simulink library "simetranss"  (R2024b)
settings: Solver=VariableStepAuto  StartTime=0.0  StopTime=10.0  RelTol=1e-3
PostLoadFcn:
  | Ts=1e-6
InitFcn:
  | Ts=1e-6
undefined symbols (not defined in the file): C, C_601, C_603, C_606, CC, Csnu, Csnubber, DiscIntNeverNeededParam, DPL, DPL1ph, FluxTable, ft2km, gcbh, h, Half, Imap2, L, L_601, L_603, L_606, Lbase, LpejoSw, Newton, R_601, R_603, R_606, Raphson, ResistanceM, Roff, Ron, RotorAngles, Rsnu, Rsnubber, Rt4, SampleTime, simetran, sps, sps_rtmsupport, StatorCurrents, T_2wind_ratio, T_Lpu, T_Lpu_pri, T_Rpu, T_Rpu_pri, T_Vpri, T_Vpri_15comp, T_Vsec, Ti, Ts_Power, Z, Zbase, Zm
libraries: fl_lib x248, ee_lib x146, nesl_utility x122, $bdroot x29, simulink x15, eeGeneralControl x2, spsStairGeneratorLib x2, artemis x1
(part 9 of 12)

== system simetranss/Machines/MATE Induction Machine/Matrice ==
  we : Inport
  park : Inport  Port=2
  0 : Constant  Value=[0 0 0 0 0 0 0 0 0 0 0 ]
  1 : Constant  Value=[0 0]
  2 : Constant  Value=0
  3 : Constant  Value=[0 0 0 0 0 0 0 0 0 0 0 ]
  4 : Constant  Value=[0 0]
  5 : Constant  Value=0
  Divide4 : Product  Multiplication=Matrix(*)
  Gain1 : Gain  Gain=1/(Lr*Ls-Lm*Lm)
  Gain3 : Gain  Gain=-1
  Gain6 : Gain
  Gain7 : Gain
  Gain8 : Gain  Gain=-1
  L-1*discriminant : Constant  Value="[Lr 0 -Lm 0; 0 Lr 0 -Lm; -Lm 0  Ls  0;  0  -Lm  0  Ls]"
  Mux1 : Mux  Inputs=[11 1 2 1 1]
  Mux2 : Mux  Inputs=[1 1 2 1 11]
  R : Constant  Value="[-Rs 0 0 0; 0 -Rs 0 0; 0 0  -Rr  0;  0  0  0  -Rr]"
  Reshape2 : Reshape  OutputDimensionality=Customize  OutputDimensions=[4,4]
  Switch : Switch  Criteria=u2 > Threshold  Threshold=0.5  SaturateOnIntegerOverflow=off  InputSameDT=off
  Adq : Outport  VectorParamsAs1DForOutWhenUnconnected=off
  invLdq : Outport  Port=2  VectorParamsAs1DForOutWhenUnconnected=off
  speed term : Outport  Port=3  VectorParamsAs1DForOutWhenUnconnected=off
  wires:
  L-1*discriminant/1 -> Gain1/1
  Reshape2/1 -> speed term/1  "OMEGA"
  R/1 -> Divide4/1
  Gain7/1 -> Mux1/2
  2/1 -> Mux1/5
  1/1 -> Mux1/3
  Divide4/1 -> Adq/1
  Gain3/1 -> Mux1/4
  0/1 -> Mux1/1
  Gain1/1 -> Divide4/2, invLdq/1  "inv(L)"
  Gain8/1 -> Mux2/2
  4/1 -> Mux2/3
  Gain6/1 -> Mux2/4
  we/1 -> Gain6/1, Gain8/1, Gain7/1, Gain3/1
  park/1 -> Switch/2
  Switch/1 -> Reshape2/1
  Mux1/1 -> Switch/1
  Mux2/1 -> Switch/3
  5/1 -> Mux2/1
  3/1 -> Mux2/5

== system simetranss/Machines/MATE Induction Machine/choose ==
  In1 : Inport
  In2 : Inport  Port=2
  In3 : Inport  Port=3
  In4 : Inport  Port=4
  In5 : Inport  Port=5
  In6 : Inport  Port=6
  In7 : Inport  Port=7
  In8 : Inport  Port=8
  In9 : Inport  Port=9
  In10 : Inport  Port=10
  Constant6 : Constant  Value=park_num
  Switch{1..5} (5 alike) : Switch  Criteria=u2 > Threshold  Threshold=0.5  SaturateOnIntegerOverflow=off  InputSameDT=off
  Out1 : Outport
  Out2 : Outport  Port=2
  Out3 : Outport  Port=3
  Out4 : Outport  Port=4
  Out5 : Outport  Port=5
  wires:
  Switch5/1 -> Out5/1
  In7/1 -> Switch2/3
  Switch4/1 -> Out4/1
  In10/1 -> Switch5/3
  In3/1 -> Switch3/1
  In5/1 -> Switch5/1
  In8/1 -> Switch3/3
  In2/1 -> Switch2/1
  In1/1 -> Switch1/1
  In6/1 -> Switch1/3
  In4/1 -> Switch4/1
  Switch2/1 -> Out2/1
  In9/1 -> Switch4/3
  Constant6/1 -> Switch1/2, Switch2/2, Switch3/2, Switch4/2, Switch5/2
  Switch1/1 -> Out1/1
  Switch3/1 -> Out3/1

== system simetranss/Machines/MATE Induction Machine/dq_fixedTransform ==
  note: Fixed reference frame
      | like rotor reference but with constant angle input=0
  Constant1 : Constant  Value=[1 -0.5 -0.5;0 sqrt(3)/2 -sqrt(3)/2]
  Gain1 : Gain  Gain=sqrt(2/3)
  Tstator : Outport  VectorParamsAs1DForOutWhenUnconnected=off
  wires:
  Constant1/1 -> Gain1/1
  Gain1/1 -> Tstator/1

== system simetranss/Machines/MATE Induction Machine/dq_rotortransform ==
  note: (rotor dq transformation reference frame)
  angle : Inport
  Enable : EnablePort
  Constant2 : Constant  Value=[1 -0.5 -0.5;0 sqrt(3)/2 -sqrt(3)/2]
  Divide : Product  Multiplication=Matrix(*)
  Gain2 : Gain  Gain=-1
  Gain4 : Gain  Gain=sqrt(2/3)
  Mux6 : Mux
  Reshape4 : Reshape  OutputDimensionality=Customize  OutputDimensions=[2,2]
  Trigonometric Function1 : Trigonometry  Operator=cos
  Trigonometric Function2 : Trigonometry
  Trotor : Outport  VectorParamsAs1DForOutWhenUnconnected=off
  wires:
  Gain4/1 -> Trotor/1  "T"
  angle/1 -> Trigonometric Function1/1, Trigonometric Function2/1
  Trigonometric Function1/1 -> Mux6/1, Mux6/4
  Trigonometric Function2/1 -> Gain2/1, Mux6/3
  Mux6/1 -> Reshape4/1
  Reshape4/1 -> Divide/1
  Constant2/1 -> Divide/2
  Divide/1 -> Gain4/1
  Gain2/1 -> Mux6/2

== system simetranss/Machines/MATE Permanent Magnet Machine (ALT1)/1 step prediction5 ==
  In1 : Inport
  Gain2 : Gain  Gain=2
  Gain3 : Gain  Gain=-1
  Sum5 : Sum  SaturateOnIntegerOverflow=on
  Unit Delay1 : UnitDelay  SampleTime=Ts  HasFrameUpgradeWarning=on
  Out1 : Outport  VectorParamsAs1DForOutWhenUnconnected=off
  wires:
  Unit Delay1/1 -> Gain3/1
  Gain2/1 -> Sum5/1
  Gain3/1 -> Sum5/2
  In1/1 -> Gain2/1, Unit Delay1/1
  Sum5/1 -> Out1/1

== system simetranss/Machines/MATE Permanent Magnet Machine (ALT1)/ABC<->dq ==
  note: (rotor dq transformation reference frame)
  angle : Inport
  Constant2 : Constant  Value=[1 -0.5 -0.5;0 sqrt(3)/2 -sqrt(3)/2]
  Divide : Product  Multiplication=Matrix(*)
  Gain2 : Gain  Gain=-1
  Gain4 : Gain  Gain=sqrt(2/3)
  Mux6 : Mux
  Reshape4 : Reshape  OutputDimensionality=Customize  OutputDimensions=[2,2]
  Trigonometric Function1 : Trigonometry  Operator=cos
  Trigonometric Function2 : Trigonometry
  T : Outport  VectorParamsAs1DForOutWhenUnconnected=off
  wires:
  Gain2/1 -> Mux6/2
  Divide/1 -> Gain4/1
  Constant2/1 -> Divide/2
  Reshape4/1 -> Divide/1
  Mux6/1 -> Reshape4/1
  Trigonometric Function2/1 -> Mux6/3, Gain2/1
  Trigonometric Function1/1 -> Mux6/4, Mux6/1
  angle/1 -> Trigonometric Function2/1, Trigonometric Function1/1
  Gain4/1 -> T/1  "T"

== system simetranss/Machines/MATE Permanent Magnet Machine (ALT1)/Bd ==
  Bc : Inport
  Product1 : Product  Multiplication=Matrix(*)  SaturateOnIntegerOverflow=on  OutDataTypeStr=Inherit: Same as first input
  trapeze has Ts/2 factor on B : Gain  Gain=Ts/2  SaturateOnIntegerOverflow=on  OutDataTypeStr=Inherit: Same as input  ParamDataTypeStr=Inherit: Same as input
  u1 : Constant  Value=Aden
  Bd : Outport  VectorParamsAs1DForOutWhenUnconnected=off
  wires:
  u1/1 -> Product1/1
  Bc/1 -> trapeze has Ts/2 factor on B/1
  trapeze has Ts/2 factor on B/1 -> Product1/2
  Product1/1 -> Bd/1

== system simetranss/Machines/MATE Permanent Magnet Machine (ALT1)/PMSM equations ==
  note: phiTot contains magnet flux
  Ad : Inport
  Bd : Inport  Port=2
  C : Inport  Port=3
  Bd_sp_term : Inport  Port=4
  C1 : Inport  Port=5
  u[n+1] : Inport  Port=6
  u_speedterm : Inport  Port=7
  fluxmagnet : Inport  Port=8
  flux_del : Inport  Port=9
  Product{1,3,5..6,8} (5 alike) : Product  Multiplication=Matrix(*)  SaturateOnIntegerOverflow=on  OutDataTypeStr=Inherit: Same as first input
  Sum1 : Sum  SaturateOnIntegerOverflow=on
  Sum2 : Sum  Inputs=+++  SaturateOnIntegerOverflow=on
  Sum3 : Sum  SaturateOnIntegerOverflow=on
  Sum5 : Sum  SaturateOnIntegerOverflow=on
  z-1 : UnitDelay  SampleTime=Ts  HasFrameUpgradeWarning=on
  z-2 : UnitDelay  SampleTime=Ts  HasFrameUpgradeWarning=on
  Ihist : Outport  VectorParamsAs1DForOutWhenUnconnected=off
  phi[n+1] : Outport  Port=2  VectorParamsAs1DForOutWhenUnconnected=off
  phiTot : Outport  Port=3  VectorParamsAs1DForOutWhenUnconnected=off
  wires:
  Bd/1 -> z-2/1
  C/1 -> Product6/1
  Product5/1 -> Sum3/1, Sum2/1
  Sum2/1 -> Product6/2, z-1/1  "Ad*phi[n]+Bd*u[n]"
  Ad/1 -> Product3/1
  u[n+1]/1 -> Product5/2
  Product3/1 -> Sum2/2
  z-1/1 -> Sum3/2
  z-2/1 -> Product5/1
  u_speedterm/1 -> Product8/2
  Bd_sp_term/1 -> Product8/1
  Product8/1 -> Sum2/3
  fluxmagnet/1 -> Sum5/2
  Sum5/1 -> phiTot/1
  Sum3/1 -> Sum5/1, phi[n+1]/1, Product3/2  "new_x"
  Product6/1 -> Sum1/1
  Sum1/1 -> Ihist/1
  Product1/1 -> Sum1/2
  C1/1 -> Product1/1
  flux_del/1 -> Product1/2

== system simetranss/Machines/MATE Permanent Magnet Machine (ALT1)/omega ==
  note: Produces: OMEGA=
      | [ 0  w ;
      | -w  0]
  In1 : Inport
  1 : Constant  Value=0
  Gain1 : Gain  Gain=-1
  Mux1 : Mux
  Reshape2 : Reshape  OutputDimensionality=Customize  OutputDimensions=[2,2]
  OMEGA : Outport
  wires:
  Reshape2/1 -> OMEGA/1  "OMEGA"
  Gain1/1 -> Mux1/2
  1/1 -> Mux1/1, Mux1/4
  Mux1/1 -> Reshape2/1
  In1/1 -> Mux1/3, Gain1/1

== system simetranss/Machines/MATE Permanent Magnet Synchronous Machine/ABC<->dq ==
  note: test for reorder block
  note: (rotor dq transformation reference frame)
  note: Derivative
  angle : Inport
  we : Inport  Port=2
  Constant : Constant  Commented=on
  Constant1 : Constant  Commented=on  Value=2
  Constant2 : Constant  Value=[1 -0.5 -0.5;0 sqrt(3)/2 -sqrt(3)/2]
  Constant3 : Constant  Commented=on  Value=3
  Constant4 : Constant  Commented=on  Value=4
  Display : Display  Commented=on
  Divide : Product  Multiplication=Matrix(*)
  Divide1 : Product  Multiplication=Matrix(*)
  Divide2 : Product
  Gain1 : Gain  Gain=sqrt(2/3)
  Gain2 : Gain  Gain=-1
  Gain3 : Gain  Gain=-1
  Gain4 : Gain  Gain=sqrt(2/3)
  Math Function3 : Math  Operator=transpose  SignedPower=on
  Mux1 : Mux
  Mux2 : Mux  Commented=on
  Mux6 : Mux
  Reshape1 : Reshape  OutputDimensionality=Customize  OutputDimensions=[2,2]
  Reshape2 : Reshape  Commented=on  OutputDimensionality=Customize  OutputDimensions=[2,2]
  Reshape4 : Reshape  OutputDimensionality=Customize  OutputDimensions=[2,2]
  Trigonometric Function1 : Trigonometry  Operator=cos
  Trigonometric Function2 : Trigonometry
  T : Outport  VectorParamsAs1DForOutWhenUnconnected=off
  dT-1/dt : Outport  Port=2  VectorParamsAs1DForOutWhenUnconnected=off
  wires:
  Reshape2/1 -> Display/1
  Mux2/1 -> Reshape2/1
  Constant4/1 -> Mux2/4
  Constant3/1 -> Mux2/3
  Constant1/1 -> Mux2/2
  Constant/1 -> Mux2/1
  we/1 -> Divide2/2
  Divide2/1 -> Gain1/1
  Divide1/1 -> Divide2/1
  Gain1/1 -> dT-1/dt/1  "T"
  Reshape1/1 -> Divide1/2
  Math Function3/1 -> Divide1/1
  Mux1/1 -> Reshape1/1
  Gain3/1 -> Mux1/3
  Gain2/1 -> Mux6/2, Mux1/4, Mux1/1  "-sin"
  Divide/1 -> Gain4/1
  Constant2/1 -> Divide/2, Math Function3/1
  Reshape4/1 -> Divide/1
  Mux6/1 -> Reshape4/1
  Trigonometric Function2/1 -> Mux6/3, Gain2/1
  Trigonometric Function1/1 -> Mux6/4, Mux6/1, Mux1/2, Gain3/1  "cos"
  angle/1 -> Trigonometric Function2/1, Trigonometric Function1/1
  Gain4/1 -> T/1  "T"

== system simetranss/Machines/MATE Synchronous Machine/1 step prediction1 ==
  In1 : Inport
  Gain2 : Gain  Gain=2
  Gain3 : Gain  Gain=-1
  Sum5 : Sum  SaturateOnIntegerOverflow=on
  Unit Delay1 : UnitDelay  SampleTime=Ts  HasFrameUpgradeWarning=on
  Out1 : Outport
  wires:
  Unit Delay1/1 -> Gain3/1
  Gain2/1 -> Sum5/1
  Gain3/1 -> Sum5/2
  In1/1 -> Gain2/1, Unit Delay1/1
  Sum5/1 -> Out1/1

== system simetranss/Machines/MATE Synchronous Machine/1 step prediction2 ==
  In1 : Inport
  Gain2 : Gain  Gain=2
  Gain3 : Gain  Gain=-1
  Sum5 : Sum  SaturateOnIntegerOverflow=on
  Unit Delay1 : UnitDelay  SampleTime=Ts  HasFrameUpgradeWarning=on
  Out1 : Outport
  wires:
  Sum5/1 -> Out1/1
  In1/1 -> Unit Delay1/1, Gain2/1
  Gain3/1 -> Sum5/2
  Gain2/1 -> Sum5/1
  Unit Delay1/1 -> Gain3/1

== system simetranss/Machines/MATE Synchronous Machine/ABC<->0 ==
  note: (homopolar transform)
  Constant2 : Constant  Value=[1 1 1]  VectorParams1D=off
  Gain4 : Gain  Gain=sqrt(1/3)
  T0 : Outport
  wires:
  Constant2/1 -> Gain4/1
  Gain4/1 -> T0/1  "T"

== system simetranss/Machines/MATE Synchronous Machine/ABC<->dq ==
  note: The Feild turn ratio gain has been moved directly in the Vfeild et IFeild signals
  note: (rotor dq transformation reference frame)
  angle : Inport
  Constant1 : Constant  Value="[0  ;0 ]"  VectorParams1D=off
  Constant2 : Constant  Value=[1 -0.5 -0.5;0 sqrt(3)/2 -sqrt(3)/2]
  Constant3 : Constant  Value=[0 0 0 Ns_on_Nf*0+1; 0 0 0 0 ; 0 0 0 0; 0 0 0 0]  VectorParams1D=off
  Divide : Product  Multiplication=Matrix(*)
  Gain2 : Gain  Gain=-1
  Gain4 : Gain  Gain=sqrt(2/3)
  Matrix Concatenate : Concatenate  Mode=Multidimensional array  ConcatenateDimension=2
  Matrix Concatenate1 : Concatenate  Mode=Multidimensional array
  Mux6 : Mux
  Reshape4 : Reshape  OutputDimensionality=Customize  OutputDimensions=[2,2]
  Selector : Selector  NumberOfDimensions=2  InputPortWidth=3  IndexOptions=Index vector (dialog),Index vector (dialog)  Indices=[1:nb_row-2],[1:4]  OutputSizes=1,1
  Trigonometric Function1 : Trigonometry  Operator=cos
  Trigonometric Function2 : Trigonometry
  T : Outport
  Tv : Outport  Port=2
  wires:
  Selector/1 -> Matrix Concatenate1/2
  angle/1 -> Trigonometric Function2/1, Trigonometric Function1/1
  Matrix Concatenate1/1 -> T/1
  Constant3/1 -> Selector/1
  Matrix Concatenate/1 -> Matrix Concatenate1/1
  Constant1/1 -> Matrix Concatenate/2
  Gain2/1 -> Mux6/2
  Divide/1 -> Gain4/1
  Constant2/1 -> Divide/2
  Reshape4/1 -> Divide/1
  Mux6/1 -> Reshape4/1
  Trigonometric Function2/1 -> Mux6/3, Gain2/1
  Trigonometric Function1/1 -> Mux6/4, Mux6/1
  Gain4/1 -> Matrix Concatenate/1, Tv/1  "T"

== system simetranss/Machines/MATE Synchronous Machine/Delta angle ==
  Vd : Inport  PortDimensions=1
  Vq : Inport  Port=2  PortDimensions=1
  Cartesian to Polar : Subsystem  mask(Cart2Polar){}
      mask help:
      | Transformation from cartesian to polar coordinates.
      | [x, y] -> [r, theta]
      |
      | r = sqrt(x^2 + y^2);
      | theta = atan(y/x);
      mask Help: Unmask this block for more help.
      mask Display: plot(0,0,100,100,[24,20,15,20,20],[85,95,85,95,20],[80,20,95,85,95,85],[70,20,20,15,20,24],[56,56,55,52,50,46],[20,26,31,35,38,42])
  Radians to Degrees : Subsystem  mask(RadiansToDegrees){}
      mask help:
      | Conversion from Radians to Degrees.
      |
      | D=180/pi*R
      mask Help: This block converts from Radians to Degrees.
      mask Display: disp('R2D')
  Terminator2 : Terminator
  delta : Outport
  wires:
  Cartesian to Polar/2(theta) -> Radians to Degrees/1(Radians in)
  Cartesian to Polar/1(r) -> Terminator2/1
  Vq/1 -> Cartesian to Polar/1(x)
  Radians to Degrees/1(Degrees out) -> delta/1  "delta"
  Vd/1 -> Cartesian to Polar/2(y)

== system simetranss/Machines/MATE Synchronous Machine/Electromagnetic Torque ==
  note: Te=phids*Iqs - phiqs*Ids
  note: Te computed from stator fluxes and currents
  phid_phiq : Inport
  id_iq : Inport  Port=2
  1-2 : Gain  Gain=[1 -1]
  Dot Product : DotProduct  OutDataTypeStr=Inherit: Inherit via internal rule
  Selector2 : Selector  InputPortWidth=2  IndexOptions=Index vector (dialog)  Indices="[2  1]"  OutputSizes=1
  Te : Outport
  wires:
  1-2/1 -> Dot Product/1
  Dot Product/1 -> Te/1
  phid_phiq/1 -> 1-2/1  "phids phiqs"
  Selector2/1 -> Dot Product/2  "iqs ids"
  id_iq/1 -> Selector2/1

== system simetranss/Machines/MATE Synchronous Machine/Phimqd ==
  note: Lad
  note: Laq
  note: phimq=  phiqs*(Laq/Ll)   +phikq1*(Laq/Llkq1)  +phikq2*(Laq/Llkq2)
      | phimd=  phids*(Lad/Ll)   +phifd*(Lad/Llfd)  + phikd*(Lad/Llkd)
  phi : Inport
  Laq : Inport  Port=2
  Lad : Inport  Port=3
  sat : Inport  Port=4
  1/Ll_d : Gain  Gain="[1/Lls   1/Llf 1/Llkd ]"  SaturateOnIntegerOverflow=on  OutDataTypeStr=Inherit: Same as input  ParamDataTypeStr=Inherit: Same as input
  1/Ll_q : Gain  Gain=[1/Lls 1/Llkq 1/Llkq2]  SaturateOnIntegerOverflow=on  OutDataTypeStr=Inherit: Same as input  ParamDataTypeStr=Inherit: Same as input
  Constant2 : Constant  Value=Lad
  Constant4 : Constant  Value=Laq
  Mux1 : Mux  Inputs=2
  Product1 : Product  RndMeth=Zero
  Product3 : Product  RndMeth=Zero
  Switch : Switch  Threshold=0.5  SaturateOnIntegerOverflow=off  InputSameDT=off
  Switch1 : Switch  Threshold=0.5  SaturateOnIntegerOverflow=off  InputSameDT=off
  "phid phifd phikd " : Selector  InputPortWidth=7  IndexOptions=Index vector (dialog)  Indices=[1 3 4]  OutputSizes=1
  phiq phikq1 (phikq2) : Selector  InputPortWidth=7  IndexOptions=Index vector (dialog)  Indices=[2 5 6]  OutputSizes=1
  sum : Sum  Inputs=+  InputSameDT=on  SaturateOnIntegerOverflow=on  OutDataTypeStr=Inherit: Same as first input
  sum1 : Sum  Inputs=+  InputSameDT=on  SaturateOnIntegerOverflow=on  OutDataTypeStr=Inherit: Same as first input
  phim_dq : Outport
  wires:
  Product1/1 -> Mux1/2  "phim_q"
  Product3/1 -> Mux1/1  "phim_d"
  "phid phifd phikd "/1 -> 1/Ll_d/1
  1/Ll_q/1 -> sum/1
  phiq phikq1 (phikq2)/1 -> 1/Ll_q/1
  phi/1 -> phiq phikq1 (phikq2)/1, "phid phifd phikd "/1
  1/Ll_d/1 -> sum1/1
  Mux1/1 -> phim_dq/1
  sum/1 -> Product1/2  "phimq"
  sum1/1 -> Product3/1  "phimd"
  Switch/1 -> Product1/1
  sat/1 -> Switch1/2, Switch/2
  Constant4/1 -> Switch/3
  Laq/1 -> Switch/1
  Constant2/1 -> Switch1/3
  Lad/1 -> Switch1/1
  Switch1/1 -> Product3/2

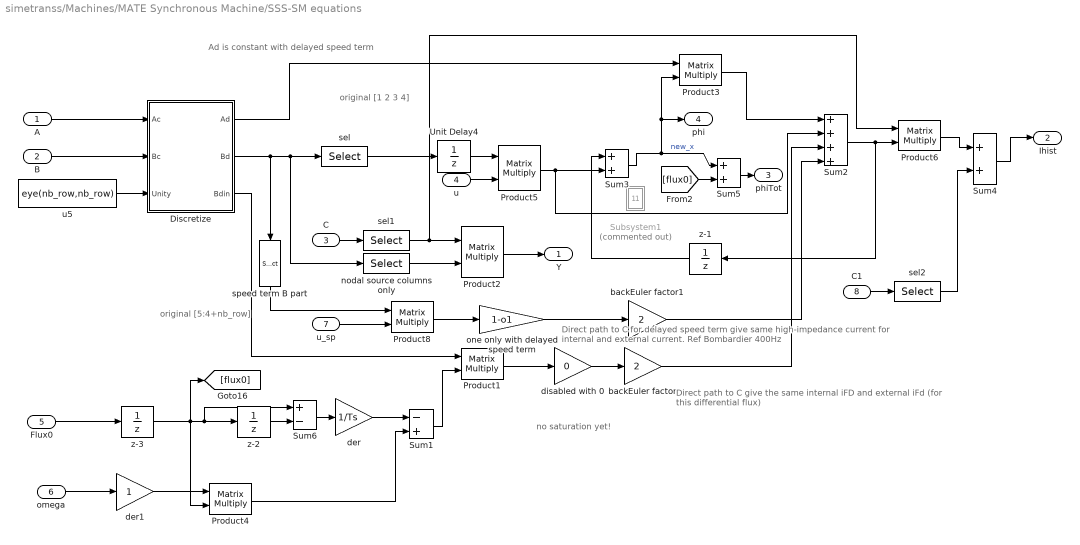
== system simetranss/Machines/MATE Synchronous Machine/SSS-SM equations ==
  note: no saturation yet!
  note: original
      | [1 2 3  4]
  note: original
      | [5:4+nb_row]
  note: Ad is constant with delayed speed term
  note: Direct path to C for delayed speed term give same high-impedance current
      | for internal and external current. Ref Bombardier 400Hz
  note: Direct path to C give the same internal iFD and external iFd
      | (for this differential flux)
  A : Inport
  B : Inport  Port=2
  C : Inport  Port=3
  u : Inport  Port=4
  Flux0 : Inport  Port=5
  omega : Inport  Port=6
  u_sp : Inport  Port=7
  C1 : Inport  Port=8
  Discretize : Subsystem
  Product{1..6,8} (7 alike) : Product  Multiplication=Matrix(*)  SaturateOnIntegerOverflow=on  OutDataTypeStr=Inherit: Same as first input
  Subsystem1 : Subsystem  Commented=on
  Sum1 : Sum  Inputs=-+  SaturateOnIntegerOverflow=on
  Sum2 : Sum  Inputs=++++  SaturateOnIntegerOverflow=on
  Sum3 : Sum  SaturateOnIntegerOverflow=on
  Sum4 : Sum  Inputs=2  SaturateOnIntegerOverflow=on
  Sum5 : Sum  SaturateOnIntegerOverflow=on
  Sum6 : Sum  Inputs=+-  SaturateOnIntegerOverflow=on
  Unit Delay4 : UnitDelay  SampleTime=Ts  HasFrameUpgradeWarning=on
  backEuler factor : Gain  Gain=2  SaturateOnIntegerOverflow=on  OutDataTypeStr=Inherit: Same as input  ParamDataTypeStr=Inherit: Same as input
  backEuler factor1 : Gain  Gain=2  SaturateOnIntegerOverflow=on  OutDataTypeStr=Inherit: Same as input  ParamDataTypeStr=Inherit: Same as input
  der : Gain  Gain=1/Ts  SaturateOnIntegerOverflow=on  OutDataTypeStr=Inherit: Same as input  ParamDataTypeStr=Inherit: Same as input
  der1 : Gain  SaturateOnIntegerOverflow=on  OutDataTypeStr=Inherit: Same as input  ParamDataTypeStr=Inherit: Same as input
  disabled with 0 : Gain  Gain=0  SaturateOnIntegerOverflow=on  OutDataTypeStr=Inherit: Same as input  ParamDataTypeStr=Inherit: Same as input
  nodal source columns only : Selector  NumberOfDimensions=2  InputPortWidth=3  IndexOptions=Index vector (dialog),Index vector (dialog)  Indices=[1:nb_row],[1 2 3]  OutputSizes=1,1
  one only with delayed speed term : Gain  Gain=1-o1
  sel : Selector  NumberOfDimensions=2  InputPortWidth=3  IndexOptions=Index vector (dialog),Index vector (dialog)  Indices="[1:nb_row],[1 2 3  ]"  OutputSizes=1,1
  sel1 : Selector  NumberOfDimensions=2  InputPortWidth=3  IndexOptions=Index vector (dialog),Index vector (dialog)  Indices=[1 2 3 ],[1:nb_row]  OutputSizes=1,1
  sel2 : Selector  InputPortWidth=4  IndexOptions=Index vector (dialog)  Indices=[1 2 3 ]  OutputSizes=1
  speed term B part : Selector  NumberOfDimensions=2  InputPortWidth=3  IndexOptions=Index vector (dialog),Index vector (dialog)  Indices=[1:nb_row],[4:3+nb_row+1]  OutputSizes=1,1
  u5 : Constant  Value=eye(nb_row,nb_row)
  z-1 : UnitDelay  InitialCondition=flux_0  SampleTime=Ts  HasFrameUpgradeWarning=on
  z-2 : UnitDelay  SampleTime=Ts  HasFrameUpgradeWarning=on
  z-3 : UnitDelay  SampleTime=Ts  HasFrameUpgradeWarning=on
  Y : Outport
  Ihist : Outport  Port=2
  phiTot : Outport  Port=3
  phi : Outport  Port=4
  wires:
  backEuler factor1/1 -> Sum2/4
  one only with delayed speed term/1 -> backEuler factor1/1
  Product8/1 -> one only with delayed speed term/1
  speed term B part/1 -> Product8/1
  u_sp/1 -> Product8/2
  sel/1 -> Unit Delay4/1
  Unit Delay4/1 -> Product5/1
  backEuler factor/1 -> Sum2/3
  Sum1/1 -> Product1/2
  der1/1 -> Product4/1
  [flux0] -> Sum5/2
  der/1 -> Sum1/1
  Product4/1 -> Sum1/2
  omega/1 -> der1/1
  Discretize/3(Bdin) -> Product1/1
  z-3/1 -> Product4/2, [flux0], Sum6/1, z-2/1
  Sum6/1 -> der/1
  z-2/1 -> Sum6/2
  Sum5/1 -> phiTot/1
  Flux0/1 -> z-3/1
  Discretize/2(Bd) -> speed term B part/1, sel/1, nodal source columns only/1
  u/1 -> Product5/2
  Discretize/1(Ad) -> Product3/1
  Sum2/1 -> Product6/2, z-1/1
  Sum3/1 -> Product3/2, phi/1, Sum5/1  "new_x"
  Product3/1 -> Sum2/1
  Product5/1 -> Sum3/2, Sum2/2
  C/1 -> sel1/1
  B/1 -> Discretize/2(Bc)
  A/1 -> Discretize/1(Ac)
  Product2/1 -> Y/1
  u5/1 -> Discretize/3(Unity)
  nodal source columns only/1 -> Product2/2
  sel1/1 -> Product6/1, Product2/1
  C1/1 -> sel2/1
  Product6/1 -> Sum4/1
  Sum4/1 -> Ihist/1
  sel2/1 -> Sum4/2
  z-1/1 -> Sum3/1
  Product1/1 -> disabled with 0/1
  disabled with 0/1 -> backEuler factor/1

== system simetranss/Machines/MATE Synchronous Machine/SSS-SM equations zero sequence only ==
  A : Inport
  B : Inport  Port=2
  C : Inport  Port=3
  u : Inport  Port=4
  Discretize : Subsystem
  Product{2..3,5..6} (4 alike) : Product  Multiplication=Matrix(*)  SaturateOnIntegerOverflow=on  OutDataTypeStr=Inherit: Same as first input
  Sum2 : Sum  SaturateOnIntegerOverflow=on
  Sum3 : Sum  SaturateOnIntegerOverflow=on
  u5 : Constant
  z-1 : UnitDelay  SampleTime=Ts  HasFrameUpgradeWarning=on
  Y0 : Outport
  Ihist0 : Outport  Port=2
  phi0 : Outport  Port=3
  wires:
  Discretize/2(Bd) -> Product2/2, Product5/1
  z-1/1 -> Sum3/1
  u/1 -> Product5/2
  Discretize/1(Ad) -> Product3/1
  Sum2/1 -> Product6/2, z-1/1
  Sum3/1 -> phi0/1, Product3/2  "new_x"
  Product3/1 -> Sum2/1
  Product5/1 -> Sum3/2, Sum2/2
  Product6/1 -> Ihist0/1
  C/1 -> Product2/1, Product6/1
  B/1 -> Discretize/2(Bc)
  A/1 -> Discretize/1(Ac)
  Product2/1 -> Y0/1
  u5/1 -> Discretize/3(Unity)

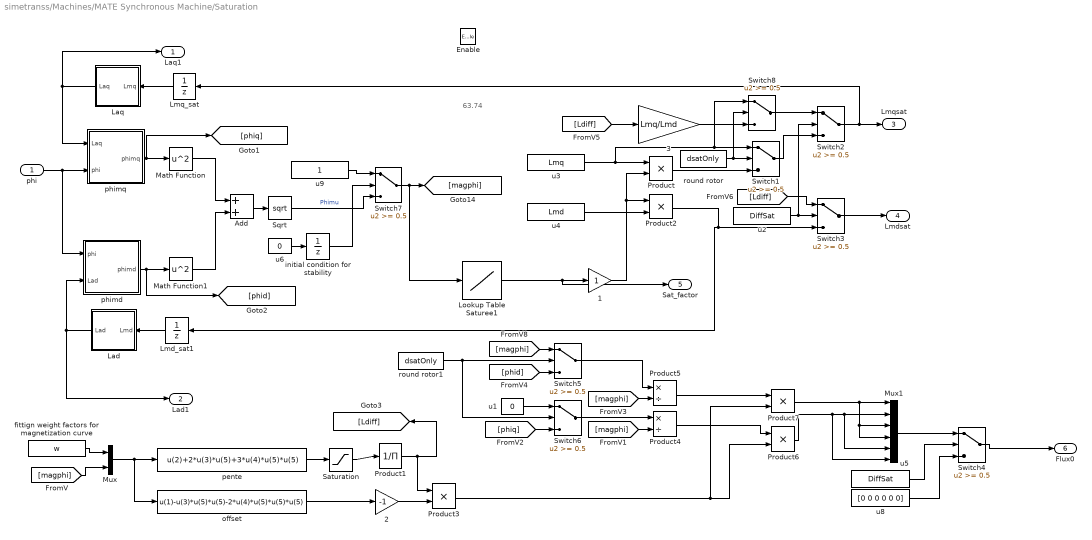
== system simetranss/Machines/MATE Synchronous Machine/Saturation ==
  note: 63.74
  phi : Inport
  Enable : EnablePort
  1 : Gain  SaturateOnIntegerOverflow=on  OutDataTypeStr=Inherit: Same as input  ParamDataTypeStr=Inherit: Same as input
  2 : Gain  Gain=-1  SaturateOnIntegerOverflow=on  OutDataTypeStr=Inherit: Same as input  ParamDataTypeStr=Inherit: Same as input
  3 : Gain  Gain=Lmq/Lmd  SaturateOnIntegerOverflow=on  OutDataTypeStr=Inherit: Same as input  ParamDataTypeStr=Inherit: Same as input
  Add : Sum
  Lad : Subsystem
  Laq : Subsystem
  Lmd_sat1 : UnitDelay  InitialCondition=Lmd  SampleTime=Ts  HasFrameUpgradeWarning=on
  Lmq_sat : UnitDelay  InitialCondition=Lmq  SampleTime=Ts  HasFrameUpgradeWarning=on
  Lookup Table Saturee1 : Lookup  InputValues=table_flux_input  Table=table_saturation_factor  SaturateOnIntegerOverflow=off
  Math Function : Math  Operator=square  SignedPower=on
  Math Function1 : Math  Operator=square  SignedPower=on
  Mux : Mux  Inputs=2
  Mux1 : Mux  Inputs=6
  Product{,2..3,6..7} (5 alike) : Product  RndMeth=Zero
  Product1 : Product  Inputs=/  RndMeth=Zero
  Product4 : Product  Inputs=*/  RndMeth=Zero
  Product5 : Product  Inputs=*/  RndMeth=Zero
  Saturation : Saturate  UpperLimit=inf  LowerLimit=1e-7
  Sqrt : Sqrt  OutputSignalType=real
  Switch{1..8} (8 alike) : Switch  Threshold=0.5  SaturateOnIntegerOverflow=off  InputSameDT=off
  fittign weight factors for magnetization curve : Constant  Value=w
  initial condition for stability : UnitDelay  InitialCondition=1  SampleTime=Ts  HasFrameUpgradeWarning=on
  offset : Fcn  Expr=u(1)-u(3)*u(5)*u(5)-2*u(4)*u(5)*u(5)*u(5)
  pente : Fcn  Expr=u(2)+2*u(3)*u(5)+3*u(4)*u(5)*u(5)
  phimd : Subsystem
  phimq : Subsystem
  round rotor : Constant  Value=dsatOnly
  round rotor1 : Constant  Value=dsatOnly
  u1 : Constant  Value=0
  u2 : Constant  Value=DiffSat
  u3 : Constant  Value=Lmq
  u4 : Constant  Value=Lmd
  u5 : Constant  Value=DiffSat
  u6 : Constant  Value=0
  u8 : Constant  Value=[0 0 0 0 0 0]
  u9 : Constant
  Laq1 : Outport
  Lad1 : Outport  Port=2
  Lmqsat : Outport  Port=3
  Lmdsat : Outport  Port=4
  Sat_factor : Outport  Port=5
  Flux0 : Outport  Port=6
  wires:
  3/1 -> Switch8/3
  Switch8/1 -> Switch2/1
  round rotor1/1 -> Switch5/2, Switch6/2
  u1/1 -> Switch6/1
  [magphi] -> Switch5/1
  Switch6/1 -> Product4/1
  Switch5/1 -> Product5/1
  [phiq] -> Switch6/3
  [phid] -> Switch5/3
  initial condition for stability/1 -> Switch7/2
  Switch7/1 -> Lookup Table Saturee1/1, [magphi]
  u9/1 -> Switch7/1
  Saturation/1 -> Product1/1
  pente/1 -> Saturation/1
  u8/1 -> Switch4/3
  u5/1 -> Switch4/2
  Switch4/1 -> Flux0/1
  Mux1/1 -> Switch4/1
  [Ldiff] -> Switch3/1
  [Ldiff] -> 3/1
  u2/1 -> Switch2/2, Switch3/2
  Switch2/1 -> Lmqsat/1, Lmq_sat/1
  Switch3/1 -> Lmdsat/1
  Product4/1 -> Product6/1
  Product5/1 -> Product7/1
  Product7/1 -> Mux1/4, Mux1/3, Mux1/1
  Product6/1 -> Mux1/6, Mux1/5, Mux1/2
  [magphi] -> Product5/2
  [magphi] -> Product4/2
  Product3/1 -> Product6/2, Product7/2
  2/1 -> Product3/2
  offset/1 -> 2/1
  Product1/1 -> Product3/1, [Ldiff]
  Mux/1 -> offset/1, pente/1
  [magphi] -> Mux/2
  fittign weight factors for magnetization curve/1 -> Mux/1
  Lookup Table Saturee1/1 -> Sat_factor/1, 1/1
  1/1 -> Product2/1, Product/2
  Switch1/1 -> Switch2/3
  Product/1 -> Switch1/3
  round rotor/1 -> Switch8/2, Switch1/2
  Lmq_sat/1 -> Laq/1(Lmq)
  phimq/1(phimq) -> Math Function/1, [phiq]
  Laq/1(Laq) -> Laq1/1, phimq/1(Laq)
  Lmd_sat1/1 -> Lad/1(Lmd)
  phimd/1(phimd) -> Math Function1/1, [phid]
  Lad/1(Lad) -> phimd/2(Lad), Lad1/1
  phi/1 -> phimq/2(phi), phimd/1(phi)
  Add/1 -> Sqrt/1
  Math Function/1 -> Add/1
  Math Function1/1 -> Add/2
  Sqrt/1 -> Switch7/3  "Phimu"
  u3/1 -> Switch8/1, Switch1/1, Product/1
  u4/1 -> Product2/2
  Product2/1 -> Switch3/3, Lmd_sat1/1
  u6/1 -> initial condition for stability/1

== system simetranss/Machines/MATE Synchronous Machine/Update Matrix L (with Lcanay) ==
  Lmq : Inport
  Lmd : Inport  Port=2
  Ll : Inport  Port=3
  Selector1 : Selector  NumberOfDimensions=2  InputPortWidth=3  IndexOptions=Index vector (dialog),Index vector (dialog)  Indices=[1:nb_row],[1:nb_row]  OutputSizes=1,1
  Selector8 : Selector  NumberOfDimensions=2  InputPortWidth=3  IndexOptions=Index vector (dialog),Index vector (dialog)  Indices=[1:nb_row],[1:nb_row]  OutputSizes=1,1
  Sum1 : Sum  SaturateOnIntegerOverflow=on
  Sum2 : Sum  SaturateOnIntegerOverflow=on
  Update Lmd rows[1] col[1] : Assignment  NumberOfDimensions=2  IndexOptions=Index vector (dialog),Index vector (dialog)  Indices=[1 3 4],[1 3 4]  OutputSizes=1,1
  "Update Lmq rows[1,5, (6)] col[1,5, (6)] " : Assignment  NumberOfDimensions=2  IndexOptions=Index vector (dialog),Index vector (dialog)  Indices=[2 5 6],[2 5 6]  OutputSizes=1,1
  u1 : Constant  Value="[0 0 0 0 0 0; 0 0 0 0 0 0; 0 0 Lcanay Lcanay 0 0; 0 0 Lcanay Lcanay 0 0; 0 0 0 0 0 0; 0 0  0 0 0 0]"
  u3 : Constant  Value=zeros(6,6)
  Lsat : Outport
  wires:
  Selector8/1 -> Update Lmd rows[1] col[1]/1
  Sum2/1 -> Lsat/1
  Ll/1 -> Sum2/2
  Lmd/1 -> Update Lmd rows[1] col[1]/2
  u3/1 -> "Update Lmq rows[1,5, (6)] col[1,5, (6)] "/1
  Lmq/1 -> "Update Lmq rows[1,5, (6)] col[1,5, (6)] "/2
  "Update Lmq rows[1,5, (6)] col[1,5, (6)] "/1 -> Selector8/1
  u1/1 -> Selector1/1
  Selector1/1 -> Sum1/2
  Update Lmd rows[1] col[1]/1 -> Sum1/1
  Sum1/1 -> Sum2/1

== system simetranss/Machines/MATE Synchronous Machine/inverse ==
  Lsat : Inport
  Enable : EnablePort
  Gain8 : Gain  Gain=-1
  Goto1 : Goto  Commented=on  GotoTag=invL
  Product3 : Product  Multiplication=Matrix(*)  SaturateOnIntegerOverflow=on  OutDataTypeStr=Inherit: Same as first input
  Rwinding : Constant  Value="[Rs 0 0 0 0 0; 0 Rs 0 0 0 0; 0 0 Rf  0 0 0; 0 0 0 Rkd 0 0; 0 0 0 0  Rkq 0; 0 0 0 0 0 Rkq2]"
  Selector8 : Selector  NumberOfDimensions=2  InputPortWidth=3  IndexOptions=Index vector (dialog),Index vector (dialog)  Indices=[1:nb_row],[1:nb_row]  OutputSizes=1,1
  inversion2 : Product  Inputs=/  Multiplication=Matrix(*)  RndMeth=Zero
  -R*inv(L) : Outport
  inv(L) : Outport  Port=2
  wires:
  Product3/1 -> -R*inv(L)/1
  Rwinding/1 -> Selector8/1
  Selector8/1 -> Gain8/1
  Lsat/1 -> inversion2/1
  inversion2/1 -> inv(L)/1, Product3/2, Goto1/1
  Gain8/1 -> Product3/1

== system simetranss/Measure/Bus Measure/Measure ==
  Kv2 : Gain  Gain=Kv  SaturateOnIntegerOverflow=on  OutDataTypeStr=Inherit: Same as input  ParamDataTypeStr=Inherit: Same as input
  Kv3 : Gain  Gain=Ki  SaturateOnIntegerOverflow=on  OutDataTypeStr=Inherit: Same as input  ParamDataTypeStr=Inherit: Same as input
  Meas : ee_lib/Sensors & Transducers/Current and Voltage Sensor (Three-Phase)  vMeasurementType=ee.enum.vmeasurement.lg  outputUnit=ee.enum.unit.si  SRated=100e6 A*V  VRated=24e3 V  I_specify=off  I_priority=None  I=[0, 0, 0] A  I_nominal_specify=off  I_nominal_value=1  I_nominal_unit=A  V_specify=off  V_priority=None  V=[0, 0, 0] V  V_nominal_specify=off  V_nominal_value=1  V_nominal_unit=V
      settings: InternalSimscapePortConfiguration="{\"Bottom\":[],\"Left\":[{\"id\":\"N1\",\"label\":\"~1\",\"type\":\"foundation.electrical.three_phase\"}],\"Right\":[{\"id\":\"V_output\",\"label\":\"V\",\"type\":\"output\"},{\"id\":\"I_output\",\"label\":\"I\",\"type\":\"output\"},{\"id\":\"N2\",\"label\":\"~2\",\"type\":\"foundation.electrical.three_phase\"}],\"Top\":[]}"
  PS-Simulink Converter : nesl_utility/PS-Simulink Converter  PhysicalDomain=network_engine_domain  SubClassName=ps_output  LeftPortType=input  RightPortType=output  PseudoPeriodic=off  Frequencies=[]  VectorFormat=inherit  Unit=inherit  AffineConversion=off
  PS-Simulink Converter1 : nesl_utility/PS-Simulink Converter  PhysicalDomain=network_engine_domain  SubClassName=ps_output  LeftPortType=input  RightPortType=output  PseudoPeriodic=off  Frequencies=[]  VectorFormat=inherit  Unit=inherit  AffineConversion=off
  Conn1 : PMIOPort  Side=Left
  Conn2 : PMIOPort  Port=2  Side=Right
  tag scope: Iabc_B1ssc=global, Vabc_B1ssc=global
  wires:
  PS-Simulink Converter1/1 -> Kv3/1
  PS-Simulink Converter/1 -> Kv2/1
  Kv2/1 -> [Vabc_B1ssc]
  Kv3/1 -> [Iabc_B1ssc]
  connections:
  Meas/RConn2 -- PS-Simulink Converter1/LConn1
  Meas/RConn1 -- PS-Simulink Converter/LConn1
  Meas/RConn3 -- Conn2/RConn1
  Meas/LConn1 -- Conn1/RConn1

== system simetranss/Measure/Bus Measure/Pass ==
  Conn1 : PMIOPort  Side=Left
  Conn2 : PMIOPort  Port=2  Side=Right
  connections:
  Conn1/RConn1 -- Conn2/RConn1

== system simetranss/Misc/Discrete Mean value/Model ==
  In : Inport
  Digital Clock : DigitalClock  SampleTime=Ts
  Discrete Variable Time Delay : Subsystem  LoadFcn=sps_rtmsupport('LoadFcn', gcbh);  StartFcn=sps_rtmsupport('StartFcn', gcbh);  StopFcn=sps_rtmsupport('StopFcn', gcbh);  mask(Discrete Variable Time Delay){MaxDelay=max(sps.Delay)+2*Ts, InitialValue=0, Ts=Ts, DFT=on}
      mask prompts: MaxDelay "Maximum delay (s):"; InitialValue "Initial conditions:"; Ts "Sample time:"; DFT "Direct feedthrough"
      mask help:
      | Apply delays (D) to the input signals (In). The block accepts a vectorized input of N signals and N delays. When the delays are not integer values of the sample time, the block interpolates.
      |
      | The initial conditions (n x N) array represents the previous input values of the N input signals:
      |     [In(-n*Ts); In(-(n-1)*Ts); ...; In(-2*Ts); In(-Ts)]
      | where:
      |     N = size of the input signals vector
      |     n = required number of previous input values (n = ceil(max(D/Ts)) at t = 0)
      |
      | When the Direct feedthrough parameter is not selected, and the time delays are lower than the sample time, the block extrapolates the inputs.
      mask init:
      | powericon('DetermineBlockChoice',gcb,Ts,0,0);
      settings: CopyFcn=sps_rtmsupport('CopyFcn', gcbh);  DeleteFcn=sps_rtmsupport('DeleteFcn', gcbh);  UndoDeleteFcn=sps_rtmsupport('UndoDeleteFcn', gcbh);  ModelCloseFcn=sps_rtmsupport('ModelCloseFcn', gcbh);  PreSaveFcn=sps_rtmsupport('PreSaveFcn', gcbh);  PostSaveFcn=sps_rtmsupport('PostSaveFcn', gcbh);  NameChangeFcn=sps_rtmsupport('NameChangeFcn', gcbh);  PreCopyFcn=sps_rtmsupport('PreCopyFcn', gcbh);  OpenFcn=sps_rtmsupport('OpenFcn', gcbh, [4]);  CloseFcn=sps_rtmsupport('CloseFcn', gcbh);  PreDeleteFcn=sps_rtmsupport('PreDeleteFcn', gcbh);
      mask Help: helpview(psbhelp);
      mask Display: disp('')
  Gain : Gain  Gain=mate.K1  SaturateOnIntegerOverflow=on  OutDataTypeStr=Inherit: Same as input  ParamDataTypeStr=Inherit: Same as input
  Gain1 : Gain  Gain=mate.K2  SaturateOnIntegerOverflow=on  OutDataTypeStr=Inherit: Same as input  ParamDataTypeStr=Inherit: Same as input
  Integ4 : DiscreteIntegrator  IntegratorMethod=Integration: Trapezoidal  SampleTime=Ts  ICPrevOutput=DiscIntNeverNeededParam  ICPrevScaledInput=DiscIntNeverNeededParam
  K1 : Constant  Value=mate.Delay  SampleTime=Ts
  K2 : Constant  Value=mate.Freq  SampleTime=Ts
  Product : Product  InputSameDT=on  SaturateOnIntegerOverflow=on  OutDataTypeStr=Inherit: Same as first input
  Relational Operator : RelationalOperator  OutDataTypeStr=boolean  SampleTime=Ts  InputSameDT=off
  Sum1 : Sum  Inputs=+-  InputSameDT=on  SaturateOnIntegerOverflow=on  OutDataTypeStr=Inherit: Same as first input
  Sum5 : Sum  InputSameDT=on  SaturateOnIntegerOverflow=on  OutDataTypeStr=Inherit: Same as first input
  Sum7 : Sum  Inputs=-+  InputSameDT=on  SaturateOnIntegerOverflow=on  OutDataTypeStr=Inherit: Same as first input
  Switch : Switch  Threshold=0.5  SaturateOnIntegerOverflow=off
  Unit Delay : UnitDelay  SampleTime=Ts  HasFrameUpgradeWarning=on
  Unit Delay1 : UnitDelay  InitialCondition=mate.Vinit  SampleTime=Ts  HasFrameUpgradeWarning=on
  Mean : Outport
  wires:
  Gain/1 -> Sum1/2
  Unit Delay/1 -> Gain/1
  Gain1/1 -> Sum1/1
  Discrete Variable Time Delay/1(Out) -> Sum7/1
  Switch/1 -> Unit Delay1/1, Mean/1
  Sum5/1 -> Switch/1
  In/1 -> Unit Delay/1, Gain1/1, Integ4/1
  K2/1 -> Product/2
  Integ4/1 -> Sum7/2, Discrete Variable Time Delay/1(In)
  Sum7/1 -> Product/1
  Product/1 -> Sum5/1  "Mean"
  Sum1/1 -> Sum5/2  "Correction"
  Unit Delay1/1 -> Switch/3
  Digital Clock/1 -> Relational Operator/1
  Relational Operator/1 -> Switch/2
  K1/1 -> Relational Operator/2, Discrete Variable Time Delay/2(D)

== system simetranss/Misc/RMS/RMS  ==
  In : Inport
  Enable : EnablePort
  Fourier : $bdroot/Misc/Fourier  Freq=mate.Freq  n=1  ParInit=mate.Par_Init_RMS  Ts=Ts
  Gain : Gain  Gain=1/sqrt(2)
  Terminator : Terminator
  RMS : Outport  VectorParamsAs1DForOutWhenUnconnected=off
  wires:
  Fourier/1 -> Gain/1
  Fourier/2 -> Terminator/1
  In/1 -> Fourier/1
  Gain/1 -> RMS/1

== system simetranss/Misc/RMS/TrueRMS  ==
  In : Inport
  Enable : EnablePort
  Discrete Mean value : $bdroot/Misc/Discrete Mean value  Freq=mate.Freq  Vinit=mate.Par_Init_TrueRMS  Ts=Ts
  Product : Product  InputSameDT=on  SaturateOnIntegerOverflow=on  OutDataTypeStr=Inherit: Same as first input
  Saturation to avoid negative sqrt : Saturate  UpperLimit=Inf  LowerLimit=0
  Sqrt : Sqrt  AlgorithmType=Newton-Raphson
  RMS : Outport  VectorParamsAs1DForOutWhenUnconnected=off
  wires:
  Saturation to avoid negative sqrt/1 -> Sqrt/1
  Discrete Mean value/1 -> Saturation to avoid negative sqrt/1
  Product/1 -> Discrete Mean value/1
  In/1 -> Product/2, Product/1
  Sqrt/1 -> RMS/1

== system simetranss/Network decoupling/MATE 3-phase Compensated Half-Stubline/Compensate ==
  Capacitor : ee_lib/Passive/Capacitor  Commented=on  cap_option=ee.enum.passive.capacitor.capOption.const  c=C_damp F  Cvec=[1e-05, 1e-06] F  Vvec=[0, 10] V  CV_table_symmetry=ee.enum.passive.capacitor.tableSymmetry.yes  f_vec=[1, 10] kHz  DFext_vec=[.8, 1.2]  enable_C_tol=ee.enum.toleranceApplication.none  averaging_period=0 s  C_tol=5  tol_distribution=ee.enum.toleranceDistribution.uniform  nSigma=4  r=0 Ohm  g=0 1/Ohm  enable_operating_limits=ee.enum.enable.no  operating_limit_action=ee.enum.passive.reportOpLim.warn  max_working_voltage_range=[-25, 25] V  power_rating=1 W  maxTemperature=85 degC  thermalEnable=false  thermalMass=1 J/K  fault_action=simscape.enum.assert.action.none  t_fault=1 s  i_specify=off  i_priority=None  i=0 A  i_nominal_specify=off  i_nominal_value=1  i_nominal_unit=A  v_specify=off  v_priority=None  v=0 V  v_nominal_specify=off  v_nominal_value=1  v_nominal_unit=V  vc_specify=off  vc_priority=High  vc=0 V  vc_nominal_specify=off  vc_nominal_value=1  vc_nominal_unit=V  T_specify=off  T_priority=None  T=298.15 K  T_nominal_specify=off  T_nominal_value=1  T_nominal_unit=K
  Capacitor1 : ee_lib/Passive/Capacitor  Commented=on  cap_option=ee.enum.passive.capacitor.capOption.const  c=C_damp F  Cvec=[1e-05, 1e-06] F  Vvec=[0, 10] V  CV_table_symmetry=ee.enum.passive.capacitor.tableSymmetry.yes  f_vec=[1, 10] kHz  DFext_vec=[.8, 1.2]  enable_C_tol=ee.enum.toleranceApplication.none  averaging_period=0 s  C_tol=5  tol_distribution=ee.enum.toleranceDistribution.uniform  nSigma=4  r=0 Ohm  g=0 1/Ohm  enable_operating_limits=ee.enum.enable.no  operating_limit_action=ee.enum.passive.reportOpLim.warn  max_working_voltage_range=[-25, 25] V  power_rating=1 W  maxTemperature=85 degC  thermalEnable=false  thermalMass=1 J/K  fault_action=simscape.enum.assert.action.none  t_fault=1 s  i_specify=off  i_priority=None  i=0 A  i_nominal_specify=off  i_nominal_value=1  i_nominal_unit=A  v_specify=off  v_priority=None  v=0 V  v_nominal_specify=off  v_nominal_value=1  v_nominal_unit=V  vc_specify=off  vc_priority=High  vc=0 V  vc_nominal_specify=off  vc_nominal_value=1  vc_nominal_unit=V  T_specify=off  T_priority=None  T=298.15 K  T_nominal_specify=off  T_nominal_value=1  T_nominal_unit=K
  Capacitor2 : ee_lib/Passive/Capacitor  Commented=on  cap_option=ee.enum.passive.capacitor.capOption.const  c=C_damp F  Cvec=[1e-05, 1e-06] F  Vvec=[0, 10] V  CV_table_symmetry=ee.enum.passive.capacitor.tableSymmetry.yes  f_vec=[1, 10] kHz  DFext_vec=[.8, 1.2]  enable_C_tol=ee.enum.toleranceApplication.none  averaging_period=0 s  C_tol=5  tol_distribution=ee.enum.toleranceDistribution.uniform  nSigma=4  r=0 Ohm  g=0 1/Ohm  enable_operating_limits=ee.enum.enable.no  operating_limit_action=ee.enum.passive.reportOpLim.warn  max_working_voltage_range=[-25, 25] V  power_rating=1 W  maxTemperature=85 degC  thermalEnable=false  thermalMass=1 J/K  fault_action=simscape.enum.assert.action.none  t_fault=1 s  i_specify=off  i_priority=None  i=0 A  i_nominal_specify=off  i_nominal_value=1  i_nominal_unit=A  v_specify=off  v_priority=None  v=0 V  v_nominal_specify=off  v_nominal_value=1  v_nominal_unit=V  vc_specify=off  vc_priority=High  vc=0 V  vc_nominal_specify=off  vc_nominal_value=1  vc_nominal_unit=V  T_specify=off  T_priority=None  T=298.15 K  T_nominal_specify=off  T_nominal_value=1  T_nominal_unit=K
  Config10 : Subsystem  mask(Unbalanced 3-phase line (pi section)){FF=FF, RR=RR, LL=LL, CC=CC, len=1}
      mask prompts: FF "Nominal frequency (Hz)"; RR "Resistance (Ohms/km)"; LL "Inductance (H/km)"; CC "Capacitance (F/km)"; len "Length (km)"
      mask help:
      | This model can be used to model unbalanced lines used in distribution grids.
      | The underlying model is a pi-line.
      mask init:
      | C11=sum(CC(1,:));
      | C22=sum(CC(2,:));
      | C33=sum(CC(3,:));
      | C12=-CC(1,2);
      | C13=-CC(1,3);
      | C23=-CC(2,3);
      mask Display:
      | plot(0,0,100,100,[20,20,80,80,90,80,80,20,20,10],[50,40,40,50,50,50,61,61,50,50],[56,39],[55,55],[44,44],[44,55],[53,50,50],[44,48,55])
      | disp(['Unbalanced \n\n 3-phase line'])
  Electrical Reference : fl_lib/Electrical/Electrical Elements/Electrical Reference  Commented=on
  Inductor : ee_lib/Passive/Inductor  Commented=on  l=L_comp H  enable_L_tol=ee.enum.toleranceApplication.none  L_tol=20  tol_distribution=ee.enum.toleranceDistribution.uniform  nSigma=4  r=0 Ohm  g=1e-9 1/Ohm  enable_operating_limits=ee.enum.enable.no  operating_limit_action=ee.enum.passive.reportOpLim.warn  max_working_current=1 A  power_rating=1 W  fault_action=simscape.enum.assert.action.none  t_fault=1 s  i_L_specify=off  i_L_priority=High  i_L=0 A  i_L_nominal_specify=off  i_L_nominal_value=1  i_L_nominal_unit=A
  Inductor1 : ee_lib/Passive/Inductor  Commented=on  l=L_comp H  enable_L_tol=ee.enum.toleranceApplication.none  L_tol=20  tol_distribution=ee.enum.toleranceDistribution.uniform  nSigma=4  r=0 Ohm  g=1e-9 1/Ohm  enable_operating_limits=ee.enum.enable.no  operating_limit_action=ee.enum.passive.reportOpLim.warn  max_working_current=1 A  power_rating=1 W  fault_action=simscape.enum.assert.action.none  t_fault=1 s  i_L_specify=off  i_L_priority=High  i_L=0 A  i_L_nominal_specify=off  i_L_nominal_value=1  i_L_nominal_unit=A
  Inductor2 : ee_lib/Passive/Inductor  Commented=on  l=L_comp H  enable_L_tol=ee.enum.toleranceApplication.none  L_tol=20  tol_distribution=ee.enum.toleranceDistribution.uniform  nSigma=4  r=0 Ohm  g=1e-9 1/Ohm  enable_operating_limits=ee.enum.enable.no  operating_limit_action=ee.enum.passive.reportOpLim.warn  max_working_current=1 A  power_rating=1 W  fault_action=simscape.enum.assert.action.none  t_fault=1 s  i_L_specify=off  i_L_priority=High  i_L=0 A  i_L_nominal_specify=off  i_L_nominal_value=1  i_L_nominal_unit=A
  Phase Splitter1 : ee_lib/Connectors & References/Phase Splitter
  Phase Splitter2 : ee_lib/Connectors & References/Phase Splitter
  Resistor : ee_lib/Passive/Resistor  Commented=on  R=R_damp Ohm  enable_R_tol=ee.enum.toleranceApplication.none  R_tol=5  tol_distribution=ee.enum.toleranceDistribution.uniform  nSigma=4  enable_operating_limits=ee.enum.enable.no  operating_limit_action=ee.enum.passive.reportOpLim.warn  power_rating=1 W  max_working_voltage=100 V  noise_mode=ee.enum.sources.noise.Disabled  Tdevice=25 degC  sample_time=1e-3 s  repeatability=ee.enum.ic.repeatability.notRepeatable  user_seed=0  auto_seed=785646024  fault_action=simscape.enum.assert.action.none  t_fault=1 s  power_derating_T1=70 degC  power_derating_T2=155 degC  operating_temperature_range_vec=[-50, 150] degC  alpha=3.93e-3 1/K  Tmeas=25 degC  thermal_mass=100 J/K  temperature_specify=off  temperature_priority=High  temperature=298.15 K  temperature_nominal_specify=off  temperature_nominal_value=1  temperature_nominal_unit=K
  Resistor1 : ee_lib/Passive/Resistor  Commented=on  R=R_damp Ohm  enable_R_tol=ee.enum.toleranceApplication.none  R_tol=5  tol_distribution=ee.enum.toleranceDistribution.uniform  nSigma=4  enable_operating_limits=ee.enum.enable.no  operating_limit_action=ee.enum.passive.reportOpLim.warn  power_rating=1 W  max_working_voltage=100 V  noise_mode=ee.enum.sources.noise.Disabled  Tdevice=25 degC  sample_time=1e-3 s  repeatability=ee.enum.ic.repeatability.notRepeatable  user_seed=0  auto_seed=1030500139  fault_action=simscape.enum.assert.action.none  t_fault=1 s  power_derating_T1=70 degC  power_derating_T2=155 degC  operating_temperature_range_vec=[-50, 150] degC  alpha=3.93e-3 1/K  Tmeas=25 degC  thermal_mass=100 J/K  temperature_specify=off  temperature_priority=High  temperature=298.15 K  temperature_nominal_specify=off  temperature_nominal_value=1  temperature_nominal_unit=K
  Resistor2 : ee_lib/Passive/Resistor  Commented=on  R=R_damp Ohm  enable_R_tol=ee.enum.toleranceApplication.none  R_tol=5  tol_distribution=ee.enum.toleranceDistribution.uniform  nSigma=4  enable_operating_limits=ee.enum.enable.no  operating_limit_action=ee.enum.passive.reportOpLim.warn  power_rating=1 W  max_working_voltage=100 V  noise_mode=ee.enum.sources.noise.Disabled  Tdevice=25 degC  sample_time=1e-3 s  repeatability=ee.enum.ic.repeatability.notRepeatable  user_seed=0  auto_seed=3807539760  fault_action=simscape.enum.assert.action.none  t_fault=1 s  power_derating_T1=70 degC  power_derating_T2=155 degC  operating_temperature_range_vec=[-50, 150] degC  alpha=3.93e-3 1/K  Tmeas=25 degC  thermal_mass=100 J/K  temperature_specify=off  temperature_priority=High  temperature=298.15 K  temperature_nominal_specify=off  temperature_nominal_value=1  temperature_nominal_unit=K
  abc. : PMIOPort  Side=Left
  abc : PMIOPort  Port=2  Side=Right
  connections:
  Capacitor2/LConn1 -- Resistor2/RConn1
  Capacitor2/RConn1 -- Capacitor1/RConn1 -- Inductor2/RConn1 -- Electrical Reference/LConn1 -- Inductor/RConn1 -- Inductor1/RConn1 -- Capacitor/RConn1
  Resistor1/RConn1 -- Capacitor1/LConn1
  Resistor/RConn1 -- Capacitor/LConn1
  Config10/RConn1 -- Inductor2/LConn1 -- Phase Splitter1/RConn1 -- Resistor2/LConn1
  Config10/RConn2 -- Inductor1/LConn1 -- Phase Splitter1/RConn2 -- Resistor1/LConn1
  Inductor/LConn1 -- Config10/RConn3 -- Resistor/LConn1 -- Phase Splitter1/RConn3
  abc./RConn1 -- Phase Splitter2/LConn1
  Phase Splitter2/RConn2 -- Config10/LConn2
  Phase Splitter2/RConn1 -- Config10/LConn1
  Phase Splitter2/RConn3 -- Config10/LConn3
  abc/RConn1 -- Phase Splitter1/LConn1

== system simetranss/Network decoupling/MATE 3-phase Compensated Half-Stubline/Pass ==
  abc. : PMIOPort  Side=Left
  abc : PMIOPort  Port=2  Side=Right
  connections:
  abc./RConn1 -- abc/RConn1
